simulink model "NMPC"  (R2024b)
settings: Solver=ode45  StartTime=0.0  StopTime=t_final  FixedStep=Ts  MaxStep=Ts  RelTol=1e-3
values from neighbouring files (symbols this model uses):
  disturbance_type = 0    [main_tilting.m]
  lin_vel_0 = [0 0 0]    [ref_trajectory.m]
  pos_0 = waypoints(1,:)    [ref_trajectory.m]
  q_0 = rotm2quat(R0)    [ref_trajectory.m]
  Ts = 0.025    [ref_trajectory.m]
  u_0 = [-params.mass*g; 0; 0; 0]    [main_tilting.m]
  w_bb_0 = [0 0 0]    [ref_trajectory.m]
undefined symbols (not defined in the file or in its folder): params
libraries: mpclib x1, robotcorelib x1, matrix_library x1, dspmathops x1
settings Model: Creator=Utente  LastModifiedBy=andreacolapinto
settings DebuggingCC: BusObjectLabelMismatch=none  UnderSpecifiedDimensionMsg=warning

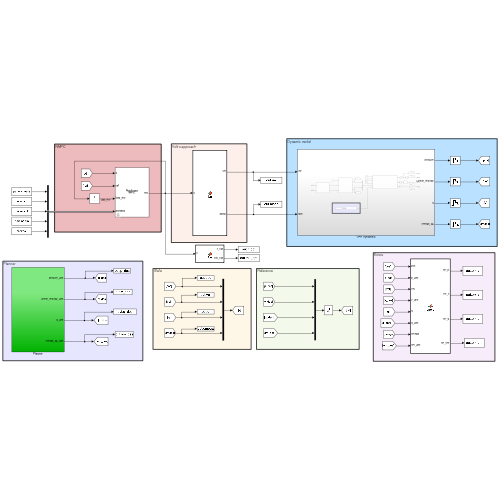
[thumbnail: Simulink's stored preview of the top-level diagram]
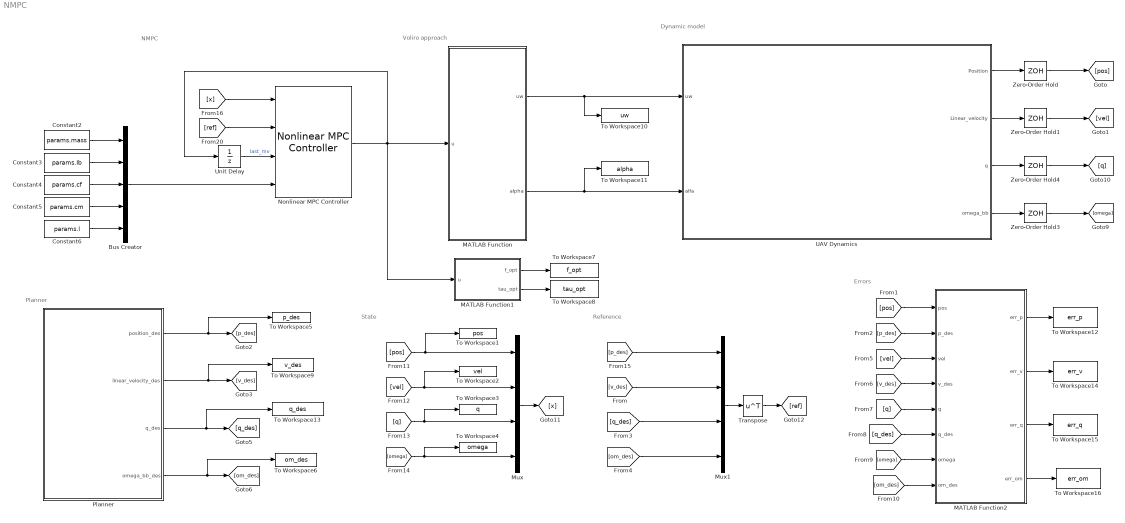
== system NMPC ==
  note: NMPC
  note: Dynamic model
  note: Voliro approach
  note: Errors
  note: Reference
  note: State
  note: Planner
  Bus Creator : BusCreator  Inputs=5  OutDataTypeStr=Bus: slBus1
  Constant2 : Constant  Value=params.mass
  Constant3 : Constant  Value=params.Ib
  Constant4 : Constant  Value=params.cf
  Constant5 : Constant  Value=params.cm
  Constant6 : Constant  Value=params.l
  MATLAB Function : MATLAB Function  TreatAsAtomicUnit=on
  MATLAB Function1 : MATLAB Function  TreatAsAtomicUnit=on
  MATLAB Function2 : MATLAB Function  TreatAsAtomicUnit=on
  Mux : Mux
  Mux1 : Mux
  Nonlinear MPC Controller : mpclib/Nonlinear MPC Controller  nlmpcobj=controller  UseObjectTs=on  UseMEX=off  mexname=UAV_model  md_enabled=off  mvtarget_enabled=off  param_enabled=on  cost_enabled=off  mvseq_enabled=off  stateseq_enabled=off  ovseq_enabled=off  slack_enabled=off  status_enabled=off  ov_min=off  ov_max=off  mv_min=off  mv_max=off  mvrate_min=off  mvrate_max=off  state_min=off  state_max=off  ov_weight=off  mv_weight=off  mvrate_weight=off  ecr_weight=off  nlp_initialize=off
  Planner : Subsystem
  To Workspace1 : ToWorkspace  VariableName=pos  SaveFormat=Structure With Time  SampleTime=-1
  To Workspace10 : ToWorkspace  VariableName=uw  SaveFormat=Structure With Time  SampleTime=-1
  To Workspace11 : ToWorkspace  VariableName=alpha  SaveFormat=Structure With Time  SampleTime=-1
  To Workspace12 : ToWorkspace  VariableName=err_p  SaveFormat=Structure With Time  SampleTime=-1
  To Workspace13 : ToWorkspace  VariableName=q_des  SaveFormat=Structure With Time  SampleTime=-1
  To Workspace14 : ToWorkspace  VariableName=err_v  SaveFormat=Structure With Time  SampleTime=-1
  To Workspace15 : ToWorkspace  VariableName=err_q  SaveFormat=Structure With Time  SampleTime=-1
  To Workspace16 : ToWorkspace  VariableName=err_om  SaveFormat=Structure With Time  SampleTime=-1
  To Workspace2 : ToWorkspace  VariableName=vel  SaveFormat=Structure With Time  SampleTime=-1
  To Workspace3 : ToWorkspace  VariableName=q  SaveFormat=Structure With Time  SampleTime=-1
  To Workspace4 : ToWorkspace  VariableName=omega  SaveFormat=Structure With Time  SampleTime=-1
  To Workspace5 : ToWorkspace  VariableName=p_des  SaveFormat=Structure With Time  SampleTime=-1
  To Workspace6 : ToWorkspace  VariableName=om_des  SaveFormat=Structure With Time  SampleTime=-1
  To Workspace7 : ToWorkspace  VariableName=f_opt  SaveFormat=Structure With Time  SampleTime=-1
  To Workspace8 : ToWorkspace  VariableName=tau_opt  SaveFormat=Structure With Time  SampleTime=-1
  To Workspace9 : ToWorkspace  VariableName=v_des  SaveFormat=Structure With Time  SampleTime=-1
  Transpose : Math  Operator=transpose
  UAV Dynamics : Subsystem
  Unit Delay : UnitDelay  InitialCondition=u_0  SampleTime=Ts  HasFrameUpgradeWarning=on
  Zero-Order Hold{,1,3..4} (4 alike) : ZeroOrderHold  SampleTime=Ts
  wires:
  Planner/4(omega_bb_des) -> To Workspace6/1, [om_des]
  Planner/3(q_des) -> To Workspace13/1, [q_des]
  Planner/2(linear_velocity_des) -> To Workspace9/1, [v_des]
  Planner/1(position_des) -> [p_des], To Workspace5/1
  UAV Dynamics/1(Position) -> Zero-Order Hold/1
  UAV Dynamics/2(Linear_velocity) -> Zero-Order Hold1/1
  UAV Dynamics/4(omega_bb) -> Zero-Order Hold3/1
  UAV Dynamics/3(q) -> Zero-Order Hold4/1
  Mux/1 -> [x]
  [x] -> Nonlinear MPC Controller/1
  [ref] -> Nonlinear MPC Controller/2
  Mux1/1 -> Transpose/1
  Transpose/1 -> [ref]
  Constant2/1 -> Bus Creator/1
  Constant3/1 -> Bus Creator/2
  Constant4/1 -> Bus Creator/3
  Constant5/1 -> Bus Creator/4
  Constant6/1 -> Bus Creator/5
  Bus Creator/1 -> Nonlinear MPC Controller/4
  Unit Delay/1 -> Nonlinear MPC Controller/3  "last_mv"
  [p_des] -> Mux1/1
  Zero-Order Hold/1 -> [pos]
  Zero-Order Hold1/1 -> [vel]
  Zero-Order Hold3/1 -> [omega]
  Zero-Order Hold4/1 -> [q]
  [v_des] -> Mux1/2
  MATLAB Function/1(uw) -> UAV Dynamics/1(uw), To Workspace10/1
  MATLAB Function/2(alpha) -> UAV Dynamics/2(alfa), To Workspace11/1
  [q_des] -> Mux1/3
  [om_des] -> Mux1/4
  [pos] -> Mux/1, To Workspace1/1
  [vel] -> To Workspace2/1, Mux/2
  [q] -> To Workspace3/1, Mux/3
  [omega] -> To Workspace4/1, Mux/4
  MATLAB Function1/1(f_opt) -> To Workspace7/1
  MATLAB Function1/2(tau_opt) -> To Workspace8/1
  [pos] -> MATLAB Function2/1(pos)
  [p_des] -> MATLAB Function2/2(p_des)
  [vel] -> MATLAB Function2/3(vel)
  [v_des] -> MATLAB Function2/4(v_des)
  [q] -> MATLAB Function2/5(q)
  [q_des] -> MATLAB Function2/6(q_des)
  [omega] -> MATLAB Function2/7(omega)
  [om_des] -> MATLAB Function2/8(om_des)
  MATLAB Function2/2(err_v) -> To Workspace14/1
  MATLAB Function2/3(err_q) -> To Workspace15/1
  MATLAB Function2/4(err_om) -> To Workspace16/1
  MATLAB Function2/1(err_p) -> To Workspace12/1
  Nonlinear MPC Controller/1 -> Unit Delay/1, MATLAB Function/1(u), MATLAB Function1/1(u)

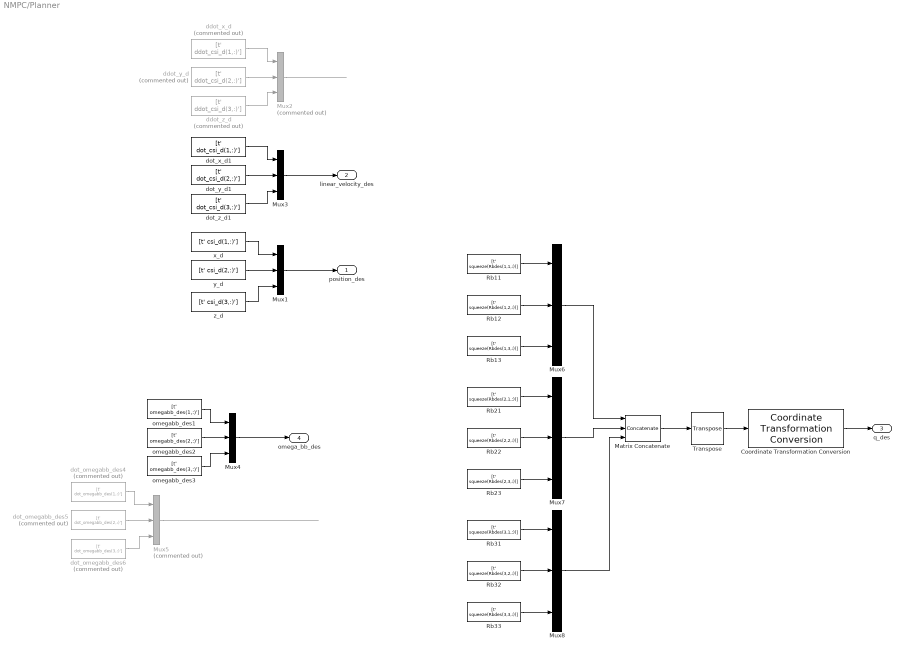
== system NMPC/Planner ==
  Coordinate Transformation Conversion : robotcorelib/Coordinate Transformation Conversion  InputRepresentation=Rotation Matrix  InputEulerSequence=ZYX  ShowTrVecInputPort=on  OutputRepresentation=Quaternion  OutputEulerSequence=ZYX  ShowTrVecOutputPort=on  SimulateUsing=Interpreted execution
  Matrix Concatenate : Concatenate  NumInputs=3  Mode=Multidimensional array  ConcatenateDimension=2
  Mux{1,3..4,6..8} (6 alike) : Mux  Inputs=3
  Mux2 : Mux  Commented=on  Inputs=3
  Mux5 : Mux  Commented=on  Inputs=3
  Rb11 : FromWorkspace  VariableName=[t' squeeze(Rbdes(1,1,:))]  SampleTime=Ts
  Rb12 : FromWorkspace  VariableName=[t' squeeze(Rbdes(1,2,:))]  SampleTime=Ts
  Rb13 : FromWorkspace  VariableName=[t' squeeze(Rbdes(1,3,:))]  SampleTime=Ts
  Rb21 : FromWorkspace  VariableName=[t' squeeze(Rbdes(2,1,:))]  SampleTime=Ts
  Rb22 : FromWorkspace  VariableName=[t' squeeze(Rbdes(2,2,:))]  SampleTime=Ts
  Rb23 : FromWorkspace  VariableName=[t' squeeze(Rbdes(2,3,:))]  SampleTime=Ts
  Rb31 : FromWorkspace  VariableName=[t' squeeze(Rbdes(3,1,:))]  SampleTime=Ts
  Rb32 : FromWorkspace  VariableName=[t' squeeze(Rbdes(3,2,:))]  SampleTime=Ts
  Rb33 : FromWorkspace  VariableName=[t' squeeze(Rbdes(3,3,:))]  SampleTime=Ts
  Transpose : matrix_library/Transpose
  ddot_x_d : FromWorkspace  Commented=on  VariableName=[t' ddot_csi_d(1,:)']  SampleTime=Ts
  ddot_y_d : FromWorkspace  Commented=on  VariableName=[t' ddot_csi_d(2,:)']  SampleTime=Ts
  ddot_z_d : FromWorkspace  Commented=on  VariableName=[t' ddot_csi_d(3,:)']  SampleTime=Ts
  dot_omegabb_des4 : FromWorkspace  Commented=on  VariableName=[t' dot_omegabb_des(1,:)']  SampleTime=Ts
  dot_omegabb_des5 : FromWorkspace  Commented=on  VariableName=[t' dot_omegabb_des(2,:)']  SampleTime=Ts
  dot_omegabb_des6 : FromWorkspace  Commented=on  VariableName=[t' dot_omegabb_des(3,:)']  SampleTime=Ts
  dot_x_d1 : FromWorkspace  VariableName=[t' dot_csi_d(1,:)']  SampleTime=Ts
  dot_y_d1 : FromWorkspace  VariableName=[t' dot_csi_d(2,:)']  SampleTime=Ts
  dot_z_d1 : FromWorkspace  VariableName=[t' dot_csi_d(3,:)']  SampleTime=Ts
  omegabb_des1 : FromWorkspace  VariableName=[t' omegabb_des(1,:)']  SampleTime=Ts
  omegabb_des2 : FromWorkspace  VariableName=[t' omegabb_des(2,:)']  SampleTime=Ts
  omegabb_des3 : FromWorkspace  VariableName=[t' omegabb_des(3,:)']  SampleTime=Ts
  x_d : FromWorkspace  VariableName=[t' csi_d(1,:)']  SampleTime=Ts
  y_d : FromWorkspace  VariableName=[t' csi_d(2,:)']  SampleTime=Ts
  z_d : FromWorkspace  VariableName=[t' csi_d(3,:)']  SampleTime=Ts
  position_des : Outport
  linear_velocity_des : Outport  Port=2
  q_des : Outport  Port=3
  omega_bb_des : Outport  Port=4
  wires:
  y_d/1 -> Mux1/2
  z_d/1 -> Mux1/3
  x_d/1 -> Mux1/1
  ddot_y_d/1 -> Mux2/2
  ddot_z_d/1 -> Mux2/3
  ddot_x_d/1 -> Mux2/1
  Mux2/1 -> ?
  Mux1/1 -> position_des/1
  dot_y_d1/1 -> Mux3/2
  dot_z_d1/1 -> Mux3/3
  dot_x_d1/1 -> Mux3/1
  Mux3/1 -> linear_velocity_des/1
  Mux5/1 -> ?
  omegabb_des3/1 -> Mux4/3
  Mux4/1 -> omega_bb_des/1
  omegabb_des2/1 -> Mux4/2
  omegabb_des1/1 -> Mux4/1
  dot_omegabb_des4/1 -> Mux5/1
  dot_omegabb_des5/1 -> Mux5/2
  dot_omegabb_des6/1 -> Mux5/3
  Rb11/1 -> Mux6/1
  Rb12/1 -> Mux6/2
  Rb13/1 -> Mux6/3
  Rb23/1 -> Mux7/3
  Rb22/1 -> Mux7/2
  Rb21/1 -> Mux7/1
  Rb31/1 -> Mux8/1
  Rb32/1 -> Mux8/2
  Rb33/1 -> Mux8/3
  Mux6/1 -> Matrix Concatenate/1
  Mux7/1 -> Matrix Concatenate/2
  Mux8/1 -> Matrix Concatenate/3
  Matrix Concatenate/1 -> Transpose/1
  Transpose/1 -> Coordinate Transformation Conversion/1
  Coordinate Transformation Conversion/1 -> q_des/1

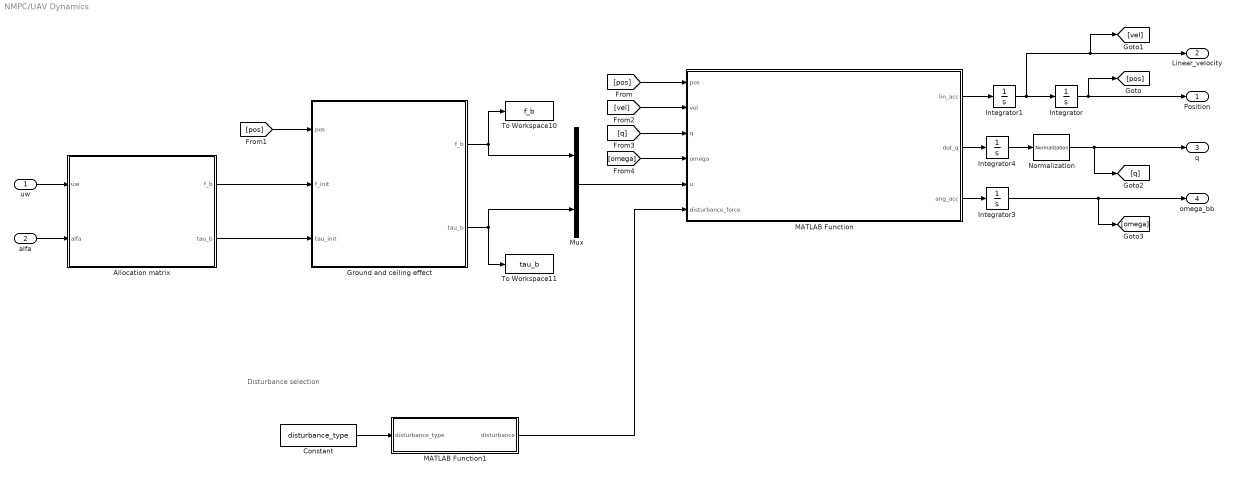
== system NMPC/UAV Dynamics ==
  note: Disturbance selection
  uw : Inport
  alfa : Inport  Port=2
  Allocation matrix : MATLAB Function  TreatAsAtomicUnit=on
  Constant : Constant  Value=disturbance_type
  Ground and ceiling effect : MATLAB Function  TreatAsAtomicUnit=on
  Integrator : Integrator  InitialCondition=pos_0'
  Integrator1 : Integrator  InitialCondition=lin_vel_0'
  Integrator3 : Integrator  InitialCondition=w_bb_0'
  Integrator4 : Integrator  InitialCondition=q_0'
  MATLAB Function : MATLAB Function  TreatAsAtomicUnit=on
  MATLAB Function1 : MATLAB Function  TreatAsAtomicUnit=on
  Mux : Mux  Inputs=2
  Normalization : dspmathops/Normalization  NormType=2-norm  Bias=1e-10  NormOver=Each column  Dimension=1  roundingMode=Floor  overflowMode=off  accumDataTypeStr=Inherit: Same as product output  accumLastDataTypeStr=Inherit: Same as product output  outputDataTypeStr=Inherit: Same as product output  outputMin=[]  outputMax=[]  outputLastDataTypeStr=Inherit: Same as product output
  To Workspace10 : ToWorkspace  VariableName=f_b  SaveFormat=Structure With Time  SampleTime=-1
  To Workspace11 : ToWorkspace  VariableName=tau_b  SaveFormat=Structure With Time  SampleTime=-1
  Position : Outport
  Linear_velocity : Outport  Port=2
  q : Outport  Port=3
  omega_bb : Outport  Port=4
  wires:
  MATLAB Function/1(lin_acc) -> Integrator1/1
  MATLAB Function/2(dot_q) -> Integrator4/1
  MATLAB Function/3(ang_acc) -> Integrator3/1
  Integrator3/1 -> [omega], omega_bb/1
  Integrator4/1 -> Normalization/1
  Normalization/1 -> [q], q/1
  alfa/1 -> Allocation matrix/2(alfa)
  uw/1 -> Allocation matrix/1(uw)
  Mux/1 -> MATLAB Function/5(u)
  Allocation matrix/1(f_b) -> Ground and ceiling effect/2(f_init)
  Allocation matrix/2(tau_b) -> Ground and ceiling effect/3(tau_init)
  Ground and ceiling effect/1(f_b) -> Mux/1, To Workspace10/1
  Ground and ceiling effect/2(tau_b) -> Mux/2, To Workspace11/1
  Integrator/1 -> [pos], Position/1
  MATLAB Function1/1(disturbance) -> MATLAB Function/6(disturbance_force)
  Constant/1 -> MATLAB Function1/1(disturbance_type)
  [pos] -> MATLAB Function/1(pos)
  [pos] -> Ground and ceiling effect/1(pos)
  Integrator1/1 -> Integrator/1, [vel], Linear_velocity/1
  [vel] -> MATLAB Function/2(vel)
  [q] -> MATLAB Function/3(q)
  [omega] -> MATLAB Function/4(omega)

== matlab function NMPC/MATLAB Function ==
  data: u input; uw output; alpha output
function [uw, alpha] = fcn(u)

cf   = 1.65776e-5;
cm   = 2.1792e-7;
l    = 0.45;

Gq = [0 0 0 -1 0 0 0 1;
    0 1 0 0 0 -1 0 0;
    -1 0 -1 0 -1 0 -1 0;
    0 0 -l -cm/cf 0 0 l cm/cf;
    l cm/cf 0 0 -l -cm/cf 0 0 ;
    -cm/cf l cm/cf -l -cm/cf l cm/cf -l];

u_=pinv(Gq)*u;

uw=zeros(4,1);
alpha=zeros(4,1);

for i= 1:4
    uw(i)=(1/cf)*sqrt(u_(2*i-1)^2+ u_(2*i)^2);
    alpha(i)=atan2(u_(2*i), u_(2*i-1));
end

== matlab function NMPC/UAV Dynamics/MATLAB Function ==
  data: pos input; vel input; q input; omega input; u input; lin_acc output; dot_q output; ang_acc output; disturbance_force input


% Dynamics
function [lin_acc, dot_q, ang_acc] = UAV_model(pos, vel, q, omega, u, disturbance_force)

mass = 1.32;
Ib   = diag([0.0154 0.0154 0.0263]);
cf   = 1.65776e-5;
cm   = 2.1792e-7;
l    = 0.45;



 mIJ=[mass*eye(3) zeros(3,3);
     zeros(3,3) Ib];

 A=[-mass*skew(omega), zeros(3,3);
     zeros(3,3) skew(Ib*omega)];



disturbance = [disturbance_force; zeros(3,1)];

% === Dinamica con disturbo ===
dyn = inv(mIJ)*(A*[vel;omega] - mass*9.81*[0 0 1 0 0 0]' + u + disturbance);

 
    lin_acc=dyn(1:3);
    ang_acc=dyn(4:6);

    % q = [q0 q1 q2 q3], omega = [wx wy wz]
qs = q(1); q1 = q(2); q2 = q(3); q3 = q(4);
wx = omega(1); wy = omega(2); wz = omega(3);

dot_q = 0.5 * [
    -q1*wx - q2*wy - q3*wz;
     qs*wx + q2*wz - q3*wy;
     qs*wy - q1*wz + q3*wx;
     qs*wz + q1*wy - q2*wx
];


end


function Gq = alloc(cf, cm, l)


Gq = [0 0 0 -1 0 0 0 1;
    0 1 0 0 0 -1 0 0;
    -1 0 -1 0 -1 0 -1 0;
    0 0 -l -cm/cf 0 0 l cm/cf;
    l cm/cf 0 0 -l -cm/cf 0 0 ;
    -cm/cf l cm/cf -l -cm/cf l cm/cf -l];


end

function S = skew(v)
    if(numel(v)~= 1)
    S= [0 -v(3) v(2); 
        v(3) 0 -v(1);
        -v(2) v(1) 0];
    else
    S= zeros(3);
    end
end

== matlab function NMPC/UAV Dynamics/Allocation matrix ==
  data: uw input size=4; alfa input size=4; f_b output size=3; tau_b output size=3
function [f_b,tau_b] = alloc_alpha(uw,alfa)

cf   = 1.65776e-5;
cm   = 2.1792e-7;
l    = 0.45;


alfa1 = alfa(1);
alfa2 = alfa(2);
alfa3 = alfa(3);
alfa4 = alfa(4);


Gq = [0 -cf*sin(alfa2) 0 cf*sin(alfa4);
    cf*sin(alfa1) 0 -cf*sin(alfa3) 0;
    -cf*cos(alfa1) -cf*cos(alfa2) -cf*cos(alfa3) -cf*cos(alfa4);
    0 -l*cf*cos(alfa2)-cm*sin(alfa2) 0 l*cf*cos(alfa4)+cm*sin(alfa4);
    l*cf*cos(alfa1)+cm*sin(alfa1) 0 -l*cf*cos(alfa3)-cm*sin(alfa3) 0;
    l*cf*sin(alfa1)-cm*cos(alfa1) -l*cf*sin(alfa2)+cm*cos(alfa2) l*cf*sin(alfa3)-cm*cos(alfa3) -l*cf*sin(alfa4)+cm*cos(alfa4)];
out = Gq*uw;
f_b = out(1:3);
tau_b = out(4:6);
end

== matlab function NMPC/UAV Dynamics/Ground and ceiling effect ==
  data: pos input size=3; f_init input size=3; tau_init input size=3; f_b output size=3; tau_b output size=3
function [f_b, tau_b] = ground_ceiling_effect(pos, f_init, tau_init)

    z = pos(3);
    rho = 0.14;
    height = 4;
    k1 = 6.924;
    k2 = 0.03782;
    
    f_b = f_init;
    tau_b = tau_init;
    
    % Ground effect
    if z > 0 && z < 2*rho
        ground_factor = 1 - (rho/(4*z))^2;
        f_b = f_init / ground_factor;
    end
    
    % Ceiling effect
    if z > height - 2*rho && z < height
        ceiling_factor = 1 - (1/k1) * ((rho/(height - z + k2))^2);
        f_b = f_b / ceiling_factor;
    end
end

== matlab function NMPC/MATLAB Function1 ==
  data: u input; f_opt output; tau_opt output
function [f_opt, tau_opt] = fcn(u)

f_opt = u(1:3);
tau_opt = u(4:6);

end

== matlab function NMPC/MATLAB Function2 ==
  data: pos input; err_p output; p_des input; vel input; v_des input; q input; q_des input; omega input; om_des input; err_v output; err_q output; err_om output
function [err_p, err_v, err_q, err_om] = errors(pos, p_des, vel, v_des, q, q_des, omega, om_des)

err_p = pos - p_des;
err_v = vel - v_des;

q = q';
q_des = q_des';
qs = q(1); qx = q(2); qy = q(3); qz = q(4);
ds = q_des(1); dx = q_des(2); dy = q_des(3); dz = q_des(4);
q_conj_s =  qs;
q_conj_x = -qx;
q_conj_y = -qy;
q_conj_z = -qz;

q_err_s = ds.*q_conj_s - dx.*q_conj_x - dy.*q_conj_y - dz.*q_conj_z;
q_err_x = ds.*q_conj_x + dx.*q_conj_s + dy.*q_conj_z - dz.*q_conj_y;
q_err_y = ds.*q_conj_y - dx.*q_conj_z + dy.*q_conj_s + dz.*q_conj_x;
q_err_z = ds.*q_conj_z + dx.*q_conj_y - dy.*q_conj_x + dz.*q_conj_s;

err_q = [q_err_s, q_err_x, q_err_y, q_err_z]';

R_err = quat2rotm(err_q');
err_om = omega - R_err*om_des;

end

== matlab function NMPC/UAV Dynamics/MATLAB Function1 ==
  data: disturbance output; disturbance_type input
function disturbance = fcn(disturbance_type)

% === Disturbo selezionabile ===

disturbance_force=zeros(3,1);

if disturbance_type == 1 
    disturbance_force = [2.5; 2.5; 0];  % costante
elseif disturbance_type == 2
    disturbance_force = 0.3 * randn(3,1);  % rumore
elseif disturbance_type == 0
    disturbance_force= zeros(3,1);
end

disturbance = disturbance_force;
